simulink model "observer"  (Simulink 8.5)
settings: Solver=ode45  StartTime=0.0  StopTime=10  RelTol=1e-3
values from neighbouring files (symbols this model uses):
  A = [0 1; 0 -c/m]    [Untitled2.m]    (also in define_consts.m; loadProperties.m; t.mat = [0  1; 0  -0.025]; test.m)
  B = [0;1/m]    [Untitled2.m]    (also in define_consts.m; loadProperties.m; t.mat = [0 0.1]; test.m = [0 0;1/m 0])
  C = [1 0]    [Untitled2.m]    (also in deadline4.m = tf([4, 1],[0, 2]); define_consts.m; loadProperties.m; t.mat)
  K = zeros(1, 2)    [createKL.m]    (also in define_consts.m; test.m = place(A,B,[p1 p2]); test_ref2.m = place(A,B,[p1(i) p2(i)]))
  k_r = K(1)    [createKL.m]    (also in define_consts.m; test_ref2.m = -1/(C*(A-B*K)^-1 *B))
  L = zeros(2, 1)    [createKL.m]    (also in define_consts.m)
  m = 7    [Untitled2.m]    (also in define_consts.m = 10; loadProperties.m = polyder(k); t.mat = 10; test.m = 10)
settings Model: Creator=Adrien  LastModifiedBy=Adrien
settings DataIOCC: SignalLoggingSaveFormat=Dataset
settings OptimizationCC: ExpressionDepthLimit=128
settings DebuggingCC: UnderspecifiedInitializationDetection=Simplified  MergeDetectMultiDrivingBlocksExec=error  FcnCallInpInsideContextMsg=EnableAllAsError  StateNameClashWarn=none
settings GRTTargetCC: CombineOutputUpdateFcns=on  GRTInterface=off

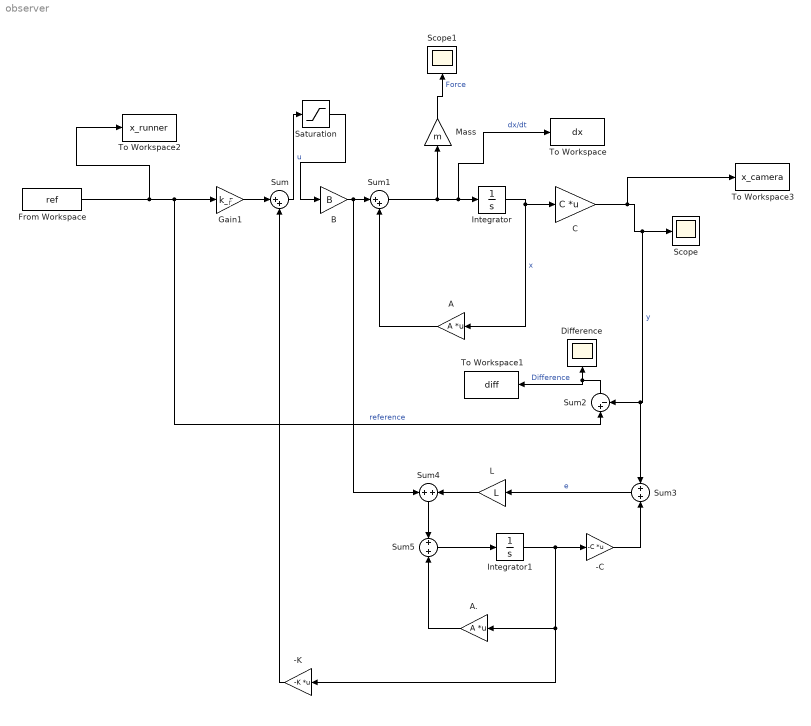
== system observer ==
  note: r
  -C : Gain  Gain=-C  Multiplication=Matrix(K*u) (u vector)
  -K : Gain  Gain=-K  Multiplication=Matrix(K*u) (u vector)
  A : Gain  Gain=A  Multiplication=Matrix(K*u) (u vector)
  A. : Gain  Gain=A  Multiplication=Matrix(K*u) (u vector)
  "B  " : Gain  Gain=B
  "C " : Gain  Gain=C  Multiplication=Matrix(K*u) (u vector)
  Difference : Scope
      settings: SaveName=ScopeData2
  From Workspace : FromWorkspace  VariableName=ref  SampleTime=step  Interpolate=off  OutputAfterFinalValue=Holding final value
  Gain1 : Gain  Gain=k_r
  Integrator : Integrator  InitialCondition=[0 0]
  Integrator1 : Integrator
  L : Gain  Gain=L
  "Mass " : Gain  Gain=m
  Saturation : Saturate  UpperLimit=70  LowerLimit=-70
  Scope : Scope
      settings: YMin=0  YMax=100
  Scope1 : Scope
  Sum : Sum  Inputs=|++
  Sum1 : Sum  Inputs=|++
  Sum2 : Sum  Inputs=|+-
  Sum3 : Sum  Inputs=+|+
  Sum4 : Sum  Inputs=+|+
  Sum5 : Sum  Inputs=+|+
  To Workspace : ToWorkspace  VariableName=dx  SaveFormat=Timeseries  SampleTime=-1
  To Workspace1 : ToWorkspace  VariableName=diff  SaveFormat=Timeseries  SampleTime=-1
  To Workspace2 : ToWorkspace  VariableName=x_runner  SaveFormat=Timeseries  SampleTime=-1
  To Workspace3 : ToWorkspace  VariableName=x_camera  SaveFormat=Timeseries  SampleTime=-1
  wires:
  Integrator/1 -> A/1, "C "/1  "x"
  "B  "/1 -> Sum4/1, Sum1/1
  A/1 -> Sum1/2
  From Workspace/1 -> Sum2/1, Gain1/1, To Workspace2/1  "reference"
  Gain1/1 -> Sum/1
  -K/1 -> Sum/2
  "C "/1 -> To Workspace3/1, Sum2/2, Sum3/1, Scope/1  "y"
  Sum1/1 -> "Mass "/1, To Workspace/1, Integrator/1  "dx/dt"
  Sum2/1 -> To Workspace1/1, Difference/1  "Difference"
  "Mass "/1 -> Scope1/1  "Force"
  Sum4/1 -> Sum5/1
  L/1 -> Sum4/2
  Sum3/1 -> L/1  "e"
  Sum5/1 -> Integrator1/1
  Integrator1/1 -> -K/1, A./1, -C/1
  -C/1 -> Sum3/2
  A./1 -> Sum5/2
  Sum/1 -> Saturation/1  "u"
  Saturation/1 -> "B  "/1
